simulink model "PD_controller_for_FODIPTD_parametric"  (R2020a)
settings: Solver=ode45  StartTime=0.0  StopTime=t_final  MaxStep=1e-3  RelTol=1e-3  EnableMultiTasking=on
undefined symbols (not defined in the file or in its folder): D, K, P, T1, tau
libraries: simulink x1
settings Model: Creator=msa  LastModifiedBy=Mohamad Chehadeh
settings DataIOCC: SaveFormat=Array  DSMLogging=off  ReturnWorkspaceOutputs=off
settings OptimizationCC: LifeSpan=inf
settings DebuggingCC: SolverPrmCheckMsg=warning  SFUnexpectedBacktrackingDiag=warning  SFNoUnconditionalDefaultTransitionDiag=warning  SFExecutionAtInitializationDiag=none  ArithmeticOperatorsInVariantConditions=warning
settings HardwareCC: ProdBitPerPointer=32  ProdBitPerSizeT=32  ProdBitPerPtrDiffT=32  ProdLargestAtomicFloat=None  ProdIntDivRoundTo=Undefined  ProdEndianess=Unspecified  ProdWordSize=32  ProdHWDeviceType=32-bit Generic
settings ModelReferenceCC: PropagateSignalLabelsOutOfModel=off
settings SFSimCC: SimUseLocalCustomCode=off  CustomCodeUndefinedFunction=UseInterfaceOnly
settings RTWCC: RTWUseLocalCustomCode=off
settings CodeAppCC: StateflowObjectComments=on
settings GRTTargetCC: TargetLangStandard=C89/C90 (ANSI)
settings ConfigComp: CovMetricSettings=dw  CovHtmlReporting=on  CovSaveCumulativeToWorkspaceVar=on  CovSaveSingleToWorkspaceVar=on  CovExternalEMLEnable=off  CovSFcnEnable=off

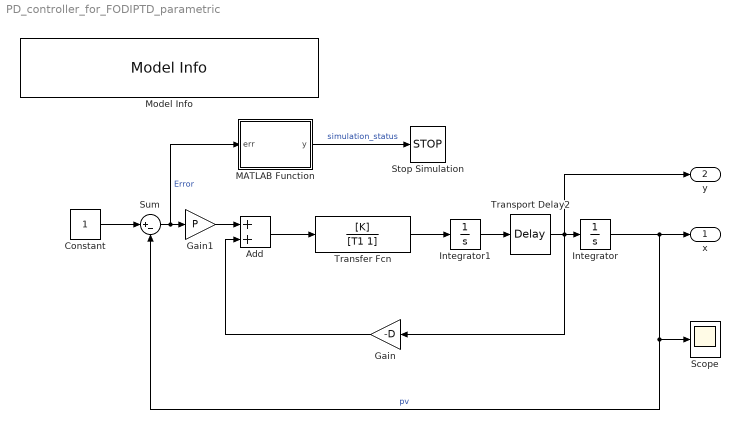
== system PD_controller_for_FODIPTD_parametric ==
  Add : Sum
  Constant : Constant
  Gain : Gain  Gain=-D
  Gain1 : Gain  Gain=P
  Integrator : Integrator
  Integrator1 : Integrator
  MATLAB Function : MATLAB Function  TreatAsAtomicUnit=on
  Model Info : simulink/Model-Wide Utilities/Model Info  Frame=on  DisplayStringWithTags=Model Info How should we take sensors reading WITHOUT delay  HorizontalTextAlignment=Center  LeftAlignmentValue=0.5
  Scope : Scope
  Stop Simulation : Stop
  Sum : Sum  Inputs=|+-
  Transfer Fcn : TransferFcn  Numerator=[K]  Denominator=[T1 1]
  Transport Delay2 : TransportDelay  DelayTime=tau
  x : Outport  VectorParamsAs1DForOutWhenUnconnected=off
  y : Outport  Port=2  VectorParamsAs1DForOutWhenUnconnected=off
  wires:
  Constant/1 -> Sum/1
  Add/1 -> Transfer Fcn/1
  Gain/1 -> Add/2
  Sum/1 -> MATLAB Function/1(err), Gain1/1  "Error"
  Integrator/1 -> Scope/1, Sum/2, x/1  "pv"
  MATLAB Function/1(y) -> Stop Simulation/1  "simulation_status"
  Transport Delay2/1 -> Gain/1, y/1, Integrator/1
  Gain1/1 -> Add/1
  Integrator1/1 -> Transport Delay2/1
  Transfer Fcn/1 -> Integrator1/1

== matlab function PD_controller_for_FODIPTD_parametric/MATLAB Function ==
  data: err input; y output
function y = fcn(err)
if (abs(err)>1000)
    y=1;
else
    y=0;
end
